simulink model "Simple_FDMA"  (Simulink 9.0)
settings: Solver=ode45  StartTime=0.0  StopTime=10.0  RelTol=1e-3  EnableMultiTasking=on
libraries: dsparch4 x6, commanapbnd3 x6, commchan3 x1
settings Model: SuppressorTable=22 serialization::archive 11 0 6 0 0 0 0 0  Creator=changgang  LastModifiedBy=changgang
settings DataIOCC: LimitDataPoints=on  SignalLoggingSaveFormat=ModelDataLogs
settings OptimizationCC: InitFltsAndDblsToZero=on
settings DebuggingCC: SaveWithParameterizedLinksMsg=none  SignalResolutionControl=TryResolveAllWithWarning  SolverPrmCheckMsg=warning  MultiTaskDSMMsg=warning  MultiTaskCondExecSysMsg=none
settings GRTTargetCC: TargetFcnLib=ansi_tfl_tmw.mat  CombineOutputUpdateFcns=off  GRTInterface=on

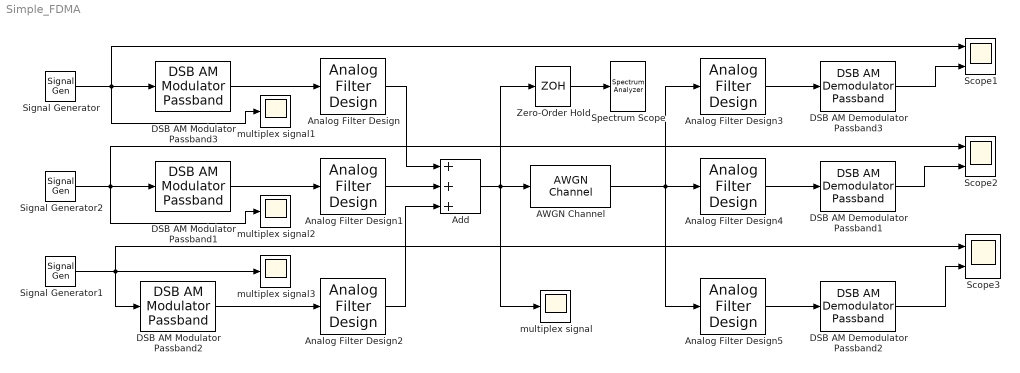
== system Simple_FDMA ==
  AWGN Channel : commchan3/AWGN Channel  InputProcessing=Inherited (this choice will be removed - see release notes)  seed=67  noiseMode=Variance from mask  EbNodB=10  EsNodB=-10  SNRdB=-10  bitsPerSym=1  Ps=1  Tsym=1  variance=0.01
  Add : Sum  Inputs=+++  SampleTime=1/320
  Analog Filter Design : dsparch4/Analog Filter Design  method=Butterworth  filttype=Bandpass  N=8  Wlo=38*2*pi  Whi=42*2*pi  Rp=2  Rs=40
  Analog Filter Design1 : dsparch4/Analog Filter Design  method=Butterworth  filttype=Bandpass  N=8  Wlo=58*2*pi  Whi=62*2*pi  Rp=2  Rs=40
  Analog Filter Design2 : dsparch4/Analog Filter Design  method=Butterworth  filttype=Bandpass  N=8  Wlo=78*2*pi  Whi=82*2*pi  Rp=2  Rs=40
  Analog Filter Design3 : dsparch4/Analog Filter Design  method=Butterworth  filttype=Bandpass  N=8  Wlo=38*2*pi  Whi=42*2*pi  Rp=2  Rs=40
  Analog Filter Design4 : dsparch4/Analog Filter Design  method=Butterworth  filttype=Bandpass  N=8  Wlo=58*2*pi  Whi=62*2*pi  Rp=2  Rs=40
  Analog Filter Design5 : dsparch4/Analog Filter Design  method=Butterworth  filttype=Bandpass  N=8  Wlo=78*2*pi  Whi=82*2*pi  Rp=2  Rs=40
  DSB AM Demodulator Passband1 : commanapbnd3/DSB AM Demodulator Passband  Fc=50  Ph=0  method=Butterworth  n=4  cf=50  Rp=0.1  Rs=50  Offset=1
      settings: SourceProductName=Communications System Toolbox  SourceProductBaseCode=CM
  DSB AM Demodulator Passband2 : commanapbnd3/DSB AM Demodulator Passband  Fc=60  Ph=0  method=Butterworth  n=4  cf=60  Rp=0.1  Rs=50  Offset=1
      settings: SourceProductName=Communications System Toolbox  SourceProductBaseCode=CM
  DSB AM Demodulator Passband3 : commanapbnd3/DSB AM Demodulator Passband  Fc=40  Ph=0  method=Butterworth  n=4  cf=40  Rp=0.1  Rs=50  Offset=1
      settings: SourceProductName=Communications System Toolbox  SourceProductBaseCode=CM
  DSB AM Modulator Passband1 : commanapbnd3/DSB AM Modulator Passband  Fc=50  Ph=0  Offset=1
      settings: SourceProductName=Communications System Toolbox  SourceProductBaseCode=CM
  DSB AM Modulator Passband2 : commanapbnd3/DSB AM Modulator Passband  Fc=60  Ph=0  Offset=1
      settings: SourceProductName=Communications System Toolbox  SourceProductBaseCode=CM
  DSB AM Modulator Passband3 : commanapbnd3/DSB AM Modulator Passband  Fc=40  Ph=0  Offset=1
      settings: SourceProductName=Communications System Toolbox  SourceProductBaseCode=CM
  Scope1 : Scope  NumInputPorts=2
  Scope2 : Scope  NumInputPorts=2
  Scope3 : Scope  NumInputPorts=2
  Signal Generator : SignalGenerator  Frequency=3  Units=rad/sec
  Signal Generator1 : SignalGenerator  Frequency=9  Units=rad/sec
  Signal Generator2 : SignalGenerator  Frequency=6  Units=rad/sec
  Spectrum Scope : SpectrumAnalyzer
  Zero-Order Hold : ZeroOrderHold  SampleTime=1/320
  multiplex signal{,1..3} (4 alike) : Scope
  wires:
  Signal Generator2/1 -> multiplex signal2/1, Scope2/1, DSB AM Modulator Passband1/1
  Signal Generator1/1 -> DSB AM Modulator Passband2/1, Scope3/1, multiplex signal3/1
  DSB AM Modulator Passband3/1 -> Analog Filter Design/1
  DSB AM Modulator Passband1/1 -> Analog Filter Design1/1
  DSB AM Modulator Passband2/1 -> Analog Filter Design2/1
  Analog Filter Design/1 -> Add/1
  Analog Filter Design1/1 -> Add/2
  Analog Filter Design2/1 -> Add/3
  Add/1 -> Zero-Order Hold/1, multiplex signal/1, AWGN Channel/1
  Zero-Order Hold/1 -> Spectrum Scope/1
  AWGN Channel/1 -> Analog Filter Design4/1, Analog Filter Design3/1, Analog Filter Design5/1
  DSB AM Demodulator Passband1/1 -> Scope2/2
  Analog Filter Design3/1 -> DSB AM Demodulator Passband3/1
  Analog Filter Design4/1 -> DSB AM Demodulator Passband1/1
  DSB AM Demodulator Passband2/1 -> Scope3/2
  Analog Filter Design5/1 -> DSB AM Demodulator Passband2/1
  DSB AM Demodulator Passband3/1 -> Scope1/2
  Signal Generator/1 -> multiplex signal1/1, Scope1/1, DSB AM Modulator Passband3/1
